simulink model "BaseEngineController_LS_112"  (Simulink 7.7)
settings: Solver=FixedStepDiscrete  StartTime=0.0  StopTime=10.0  RelTol=1e-3
PreLoadFcn:
  | try, eval([bdroot '_setup']); catch, eval('model_setup', ''); end
InitFcn:
  | try, eval([bdroot '_setup']); catch, eval('model_setup', ''); end
undefined symbols (not defined in the file): ECM, H1, H2, High, motohawk_build_version, motohawk_trunc_name, motohawk_vardec_config_group, motohawk_vardec_path, True, xD
libraries: MotoHawk_lib x1417, motohawk_control_primitives_lib x183, motohawk_engine_lib x32, simulink x21, motohawk_annotations_lib x9, AutoDoc_lib x8, simulink_extras x4, motohawk_ccp_examples_lib x1, motohawk_control_primitives_motoshare_lib x1
(part 5 of 27)

== system BaseEngineController_LS_112/Foreground/Control/Controller/Stall ==
  Inputs : Inport
  Enable : EnablePort  StatesWhenEnabling=reset
  Bus Creator2 : BusCreator  Inputs=13
  Data Type Conversion : DataTypeConversion  OutDataTypeStr=double
  Data Type Conversion1 : DataTypeConversion  OutDataTypeStr=double
  Data Type Conversion2 : DataTypeConversion  OutDataTypeStr=double
  FAN Control : Subsystem
  Fuel Pump at Startup : Subsystem
  No Fuel : Constant  Value=0
  No Spark : Constant  Value=0  OutDataTypeStr=Inherit: Inherit via back propagation
  No Spark Timing : Constant  Value=0  OutDataTypeStr=Inherit: Inherit via back propagation
  No Start EOI : Constant  Value=0
  No Start Fuel Timing : Constant  Value=0
  OFF{,1..3} (4 alike) : Constant  Value=0  OutDataTypeStr=boolean
  Stall Throttle : Subsystem
  Zero-Order Hold{1..9,11..14} (13 alike) : ZeroOrderHold  SampleTime=-1
  motohawk_replicate : MotoHawk_lib/Extra Development Blocks/motohawk_replicate  output_width=-1
  motohawk_replicate2 : MotoHawk_lib/Extra Development Blocks/motohawk_replicate  output_width=-1
  Actuators : Outport
  wires:
  Zero-Order Hold6/1 -> Bus Creator2/1  "FPC"
  No Spark/1 -> Zero-Order Hold4/1
  No Spark Timing/1 -> motohawk_replicate2/1
  No Fuel/1 -> motohawk_replicate/1
  Zero-Order Hold8/1 -> Bus Creator2/2  "SOI"
  No Start Fuel Timing/1 -> Zero-Order Hold8/1
  Bus Creator2/1 -> Actuators/1
  Stall Throttle/1(ETC %) -> Zero-Order Hold9/1
  Zero-Order Hold4/1 -> Bus Creator2/4  "SparkEnergy"
  Zero-Order Hold3/1 -> Bus Creator2/5  "SparkAdv"
  Zero-Order Hold9/1 -> Bus Creator2/6  "Throttle"
  Zero-Order Hold7/1 -> Bus Creator2/7  "FUELP"
  motohawk_replicate/1 -> Zero-Order Hold6/1
  Zero-Order Hold5/1 -> Bus Creator2/3  "EOI"
  No Start EOI/1 -> Zero-Order Hold5/1
  motohawk_replicate2/1 -> Zero-Order Hold3/1
  Fuel Pump at Startup/1(FUELP [bool]) -> Zero-Order Hold7/1
  OFF2/1 -> Zero-Order Hold1/1
  Zero-Order Hold1/1 -> Data Type Conversion2/1  "IAC-P"
  Zero-Order Hold2/1 -> Data Type Conversion1/1  "IAC-S"
  OFF/1 -> Zero-Order Hold11/1
  Zero-Order Hold11/1 -> Data Type Conversion/1  "WASTEGATE"
  OFF1/1 -> Zero-Order Hold2/1
  FAN Control/1(FAN-1) -> Zero-Order Hold12/1
  FAN Control/2(FAN-2) -> Zero-Order Hold13/1
  Inputs/1 -> FAN Control/1(Sensors), Stall Throttle/1(Sensors)
  OFF3/1 -> Zero-Order Hold14/1
  Data Type Conversion2/1 -> Bus Creator2/8  "IAC-P"
  Data Type Conversion1/1 -> Bus Creator2/9  "IAC-S"
  Data Type Conversion/1 -> Bus Creator2/10  "WASTEGATE"
  Zero-Order Hold12/1 -> Bus Creator2/11  "FAN-1"
  Zero-Order Hold13/1 -> Bus Creator2/12  "FAN-2"
  Zero-Order Hold14/1 -> Bus Creator2/13  "AC"

== system BaseEngineController_LS_112/Foreground/Control/Diagnostics/AC Fault ==
  Sensors : Inport
  Controller : Inport  Port=2
  Bus Selector1 : BusSelector  OutputSignals=Raw.LinearSensors.ACPres
  Bus Selector2 : BusSelector  OutputSignals=AC
  Logical Operator : Logic  Inputs=3  AllPortsSameDT=off  OutDataTypeStr=boolean
  Logical Operator1 : Logic  Inputs=4  AllPortsSameDT=off  OutDataTypeStr=boolean
  Logical Operator3 : Logic  Operator=OR  AllPortsSameDT=off  OutDataTypeStr=boolean
  Logical Operator4 : Logic  Operator=NOT  Inputs=3  AllPortsSameDT=off  OutDataTypeStr=boolean
  Relational Operator : RelationalOperator  OutDataTypeStr=boolean
  Relational Operator1 : RelationalOperator  Operator=<=  OutDataTypeStr=boolean
  Run State : motohawk_control_primitives_lib/CompareTo  SystemSampleTime=-1  op===  val=3
  motohawk_calibration : MotoHawk_lib/Calibration & Probing Blocks/motohawk_calibration  nam='ACHighPressureDisable'  val=3000  storage=Calibration  show_more=on  name_source=Use Parameter  data_type=uint16  read_level=1  write_level=1  ovr_cals=on  view_as=Number  enum_struct={'Disabled', 'Enabled'}  vector_style=Wide Row  use_help_units=on  help='Pressure when ac gets disabled'  units='kpa'  use_header_enum=off  row_header_enum={}  col_header_enum={}  use_min_max=off  min_val=-inf  max_val=inf  use_precision=off  precision=''  gain=1  offset=0  exp=1  use_mototune_group=off  mototune_group=motohawk_vardec_path(gcb)
  motohawk_calibration2 : MotoHawk_lib/Calibration & Probing Blocks/motohawk_calibration  nam='ACLowPressureDisable'  val=300  storage=Calibration  show_more=on  name_source=Use Parameter  data_type=uint16  read_level=1  write_level=1  ovr_cals=on  view_as=Number  enum_struct={'Disabled', 'Enabled'}  vector_style=Wide Row  use_help_units=on  help='Pressure when ac gets disabled'  units='kpa'  use_header_enum=off  row_header_enum={}  col_header_enum={}  use_min_max=off  min_val=-inf  max_val=inf  use_precision=off  precision=''  gain=1  offset=0  exp=1  use_mototune_group=off  mototune_group=motohawk_vardec_path(gcb)
  motohawk_data_read : MotoHawk_lib/Data Storage Blocks/motohawk_data_read  source=Lookup By Name  structure=Scalar  operation=Read entire data structure at once  sz_vec=4  sz_row=2  sz_col=3  typ=uint8  nam='EngineState'  checkNull=on  struct_inst_name='Struct1'  struct_nam='MyStruct'
  motohawk_fault_def1 : MotoHawk_lib/Fault Management Blocks/motohawk_fault_def  nam='ACChargeHigh_Fault'  mode=Enabled  id=[]  x=25  y=50  input_suspected=on  indeterminate=off  increment_xy=on  downsample_count=1  ovr_cals=on  ovr_actions=on  show_actions=on  action1_name='DisableAC'  action1_cond=Active  action2_name=''  action2_cond=(None)  action3_name=''  action3_cond=(None)  action4_name=''  action4_cond=(None)
  motohawk_fault_def2 : MotoHawk_lib/Fault Management Blocks/motohawk_fault_def  nam='ACChargeLow_Fault'  mode=Enabled  id=[]  x=25  y=50  input_suspected=on  indeterminate=off  increment_xy=on  downsample_count=1  ovr_cals=on  ovr_actions=on  show_actions=on  action1_name='DisableAC'  action1_cond=Active  action2_name=''  action2_cond=(None)  action3_name=''  action3_cond=(None)  action4_name=''  action4_cond=(None)
  motohawk_fault_status1 : MotoHawk_lib/Fault Management Blocks/motohawk_fault_status  source=Lookup By Name  nam='ACPresRangeHigh'  status=Active
  motohawk_fault_status4 : MotoHawk_lib/Fault Management Blocks/motohawk_fault_status  source=Lookup By Name  nam='ACPresRangeLow'  status=Active
  wires:
  Sensors/1 -> Bus Selector1/1
  motohawk_data_read/1 -> Run State/1
  Logical Operator/1 -> motohawk_fault_def1/1
  Logical Operator1/1 -> motohawk_fault_def2/1
  Controller/1 -> Bus Selector2/1
  Relational Operator/1 -> Logical Operator/2
  Bus Selector1/1 -> Relational Operator/1, Relational Operator1/1  "<ACPres>"
  motohawk_calibration/1 -> Relational Operator/2
  motohawk_calibration2/1 -> Relational Operator1/2
  Relational Operator1/1 -> Logical Operator1/2
  motohawk_fault_status1/1 -> Logical Operator3/1
  Logical Operator3/1 -> Logical Operator4/1
  motohawk_fault_status4/1 -> Logical Operator3/2
  Bus Selector2/1 -> Logical Operator1/4  "<AC>"
  Run State/1 -> Logical Operator/1, Logical Operator1/1
  Logical Operator4/1 -> Logical Operator/3, Logical Operator1/3

== system BaseEngineController_LS_112/Foreground/Control/Diagnostics/AirFlow ==
  Sensors : Inport
  Abs : Abs
  Bus Selector1 : BusSelector  OutputSignals=RawIndexes.RPM09Idx,RawIndexes.MAP09Idx
  Bus Selector4 : BusSelector  OutputSignals=Raw.Digital.MAF
  Logical Operator1 : Logic  Operator=NOT  Inputs=3  AllPortsSameDT=off  OutDataTypeStr=boolean
  Logical Operator2 : Logic  Operator=OR  Inputs=4  AllPortsSameDT=off  OutDataTypeStr=boolean
  Logical Operator3 : Logic  Operator=OR  Inputs=4  AllPortsSameDT=off  OutDataTypeStr=boolean
  Logical Operator4 : Logic  Inputs=3  AllPortsSameDT=off  OutDataTypeStr=boolean
  Logical Operator5 : Logic  Operator=OR  Inputs=3  AllPortsSameDT=off  OutDataTypeStr=boolean
  Logical Operator6 : Logic  Operator=NOT  Inputs=3  AllPortsSameDT=off  OutDataTypeStr=boolean
  Logical Operator7 : Logic  AllPortsSameDT=off  OutDataTypeStr=boolean
  Logical Operator8 : Logic  Inputs=3  AllPortsSameDT=off  OutDataTypeStr=boolean
  Logical Operator9 : Logic  Operator=NOT  Inputs=3  AllPortsSameDT=off  OutDataTypeStr=boolean
  Relational Operator : RelationalOperator  OutDataTypeStr=boolean
  Run State : motohawk_control_primitives_lib/CompareTo  SystemSampleTime=-1  op===  val=3
  Sum : Sum  Inputs=|+-
  motohawk_calibration3 : MotoHawk_lib/Calibration & Probing Blocks/motohawk_calibration  nam='AirflowDiag_MAPIRDiagEnable'  val=0  storage=Calibration  show_more=on  name_source=Use Parameter  data_type=boolean  read_level=1  write_level=1  ovr_cals=on  view_as=Enumeration  enum_struct={'Disabled', 'Enabled'}  vector_style=Wide Row  use_help_units=off  help=''  units=''  use_header_enum=off  row_header_enum={}  col_header_enum={}  use_min_max=off  min_val=-inf  max_val=inf  use_precision=off  precision=''  gain=1  offset=0  exp=1  use_mototune_group=off  mototune_group=motohawk_vardec_path(gcb)
  motohawk_data_read : MotoHawk_lib/Data Storage Blocks/motohawk_data_read  source=Lookup By Name  structure=Scalar  operation=Read scalar from location by index  sz_vec=4  sz_row=2  sz_col=3  typ=double  nam='VEModelMAF'  checkNull=on  struct_inst_name='MyData'  struct_nam='MyStruct'
  motohawk_data_read1 : MotoHawk_lib/Data Storage Blocks/motohawk_data_read  source=Lookup By Name  structure=Scalar  operation=Read entire data structure at once  sz_vec=4  sz_row=2  sz_col=3  typ=uint8  nam='EngineState'  checkNull=on  struct_inst_name='Struct1'  struct_nam='MyStruct'
  motohawk_fault_def1 : MotoHawk_lib/Fault Management Blocks/motohawk_fault_def  nam='AirflowMismatch_Fault'  mode=Enabled  id=[]  x=25  y=50  input_suspected=on  indeterminate=off  increment_xy=on  downsample_count=1  ovr_cals=on  ovr_actions=on  show_actions=on  action1_name=''  action1_cond=(None)  action2_name=''  action2_cond=(None)  action3_name=''  action3_cond=(None)  action4_name=''  action4_cond=(None)
  motohawk_fault_status1 : MotoHawk_lib/Fault Management Blocks/motohawk_fault_status  source=Lookup By Name  nam='MAPRangeHigh'  status=Active
  motohawk_fault_status10 : MotoHawk_lib/Fault Management Blocks/motohawk_fault_status  source=Lookup By Name  nam='CamSyncFault'  status=Active
  motohawk_fault_status11 : MotoHawk_lib/Fault Management Blocks/motohawk_fault_status  source=Lookup By Name  nam='CrankEdgesFault'  status=Active
  motohawk_fault_status2 : MotoHawk_lib/Fault Management Blocks/motohawk_fault_status  source=Lookup By Name  nam='MAP_IR_HI'  status=Active
  motohawk_fault_status3 : MotoHawk_lib/Fault Management Blocks/motohawk_fault_status  source=Lookup By Name  nam='MAP_IR_LO'  status=Active
  motohawk_fault_status4 : MotoHawk_lib/Fault Management Blocks/motohawk_fault_status  source=Lookup By Name  nam='MAPRangeLow'  status=Active
  motohawk_fault_status5 : MotoHawk_lib/Fault Management Blocks/motohawk_fault_status  source=Lookup By Name  nam='MAP_STICKING'  status=Active
  motohawk_fault_status6 : MotoHawk_lib/Fault Management Blocks/motohawk_fault_status  source=Lookup By Name  nam='MAFRangeHigh'  status=Active
  motohawk_fault_status7 : MotoHawk_lib/Fault Management Blocks/motohawk_fault_status  source=Lookup By Name  nam='MAFRangeLow'  status=Active
  motohawk_fault_status8 : MotoHawk_lib/Fault Management Blocks/motohawk_fault_status  source=Lookup By Name  nam='CrankSyncFault'  status=Active
  motohawk_fault_status9 : MotoHawk_lib/Fault Management Blocks/motohawk_fault_status  source=Lookup By Name  nam='CamEdgesFault'  status=Active
  motohawk_interpolation_2d : MotoHawk_lib/Lookup Tables/motohawk_interpolation_2d  nam='AirflowMimatchThresh'  table_data=zeros(9,9)  show_more=on  data_type=int8  storage=NonAdaptive  read_level=1  write_level=1  ovr_cals=on  use_help=off  help=''  units=''  use_min_max=off  min_val=-inf  max_val=inf  use_precision=off  precision=''  gain=1  offset=0  exp=1  use_links=off  row_prelookup_block=''  col_prelookup_block=''  output_name=''  use_mototune_group=off  mototune_group=motohawk_vardec_path(gcb)
  wires:
  Sensors/1 -> Bus Selector4/1, Bus Selector1/1
  motohawk_data_read1/1 -> Run State/1
  Run State/1 -> Logical Operator4/3
  Logical Operator4/1 -> motohawk_fault_def1/1
  Bus Selector4/1 -> Sum/1  "<MAF>"
  motohawk_data_read/1 -> Sum/2
  Sum/1 -> Abs/1
  Abs/1 -> Relational Operator/1
  Bus Selector1/1 -> motohawk_interpolation_2d/1  "<RPM09Idx>"
  Bus Selector1/2 -> motohawk_interpolation_2d/2  "<MAP09Idx>"
  motohawk_interpolation_2d/1 -> Relational Operator/2
  Relational Operator/1 -> Logical Operator4/2
  motohawk_fault_status1/1 -> Logical Operator3/1
  Logical Operator3/1 -> Logical Operator1/1
  motohawk_fault_status4/1 -> Logical Operator3/2
  motohawk_fault_status2/1 -> Logical Operator5/1
  motohawk_fault_status3/1 -> Logical Operator5/2
  motohawk_fault_status5/1 -> Logical Operator5/3
  Logical Operator5/1 -> Logical Operator7/1
  motohawk_calibration3/1 -> Logical Operator7/2
  Logical Operator7/1 -> Logical Operator6/1
  Logical Operator1/1 -> Logical Operator8/1
  Logical Operator6/1 -> Logical Operator8/2
  motohawk_fault_status6/1 -> Logical Operator3/3
  motohawk_fault_status7/1 -> Logical Operator3/4
  motohawk_fault_status8/1 -> Logical Operator2/1
  Logical Operator2/1 -> Logical Operator9/1
  motohawk_fault_status11/1 -> Logical Operator2/2
  motohawk_fault_status9/1 -> Logical Operator2/3
  motohawk_fault_status10/1 -> Logical Operator2/4
  Logical Operator9/1 -> Logical Operator8/3
  Logical Operator8/1 -> Logical Operator4/1

== system BaseEngineController_LS_112/Foreground/Control/Diagnostics/Boost Fault ==
  note: BOOST Level
  Sensors : Inport
  Controller : Inport  Port=2
  Bus Selector1 : BusSelector  OutputSignals=Raw.LinearSensors.MAP_Angular
  Bus Selector2 : BusSelector  OutputSignals=WASTEGATE
  Logical Operator : Logic  Inputs=3  AllPortsSameDT=off  OutDataTypeStr=boolean
  Logical Operator1 : Logic  Inputs=3  AllPortsSameDT=off  OutDataTypeStr=boolean
  Logical Operator2 : Logic  Inputs=3  AllPortsSameDT=off  OutDataTypeStr=boolean
  Logical Operator3 : Logic  Operator=OR  AllPortsSameDT=off  OutDataTypeStr=boolean
  Logical Operator4 : Logic  Operator=NOT  Inputs=3  AllPortsSameDT=off  OutDataTypeStr=boolean
  Logical Operator5 : Logic  Operator=OR  Inputs=3  AllPortsSameDT=off  OutDataTypeStr=boolean
  Logical Operator6 : Logic  Operator=NOT  Inputs=3  AllPortsSameDT=off  OutDataTypeStr=boolean
  Logical Operator7 : Logic  AllPortsSameDT=off  OutDataTypeStr=boolean
  Logical Operator8 : Logic  AllPortsSameDT=off  OutDataTypeStr=boolean
  Relational Operator : RelationalOperator  OutDataTypeStr=boolean
  Relational Operator1 : RelationalOperator  OutDataTypeStr=boolean
  Relational Operator2 : RelationalOperator  OutDataTypeStr=boolean
  Run State : motohawk_control_primitives_lib/CompareTo  SystemSampleTime=-1  op===  val=3
  kPa to PSI : Gain  Gain=0.145038
  motohawk_calibration : MotoHawk_lib/Calibration & Probing Blocks/motohawk_calibration  nam='SoftOverBoostLimit'  val=20  storage=Calibration  show_more=on  name_source=Use Parameter  data_type=Inherit from 'Default Value'  read_level=1  write_level=1  ovr_cals=on  view_as=Number  enum_struct={'Disabled', 'Enabled'}  vector_style=Wide Row  use_help_units=on  help='Soft overboost limit'  units='PSI'  use_header_enum=off  row_header_enum={}  col_header_enum={}  use_min_max=off  min_val=-inf  max_val=inf  use_precision=off  precision=''  gain=1  offset=0  exp=1  use_mototune_group=off  mototune_group=motohawk_vardec_path(gcb)
  motohawk_calibration1 : MotoHawk_lib/Calibration & Probing Blocks/motohawk_calibration  nam='HardOverBoostLimit'  val=25  storage=Calibration  show_more=on  name_source=Use Parameter  data_type=Inherit from 'Default Value'  read_level=1  write_level=1  ovr_cals=on  view_as=Number  enum_struct={'Disabled', 'Enabled'}  vector_style=Wide Row  use_help_units=on  help='Hard overboost limit'  units='PSI'  use_header_enum=off  row_header_enum={}  col_header_enum={}  use_min_max=off  min_val=-inf  max_val=inf  use_precision=off  precision=''  gain=1  offset=0  exp=1  use_mototune_group=off  mototune_group=motohawk_vardec_path(gcb)
  motohawk_calibration2 : MotoHawk_lib/Calibration & Probing Blocks/motohawk_calibration  nam='WastegateLossOfControl'  val=50  storage=Calibration  show_more=on  name_source=Use Parameter  data_type=Inherit from 'Default Value'  read_level=1  write_level=1  ovr_cals=on  view_as=Number  enum_struct={'Disabled', 'Enabled'}  vector_style=Wide Row  use_help_units=on  help='Wastegate duty cycle having insufficient control of boost'  units='%'  use_header_enum=off  row_header_enum={}  col_header_enum={}  use_min_max=off  min_val=-inf  max_val=inf  use_precision=off  precision=''  gain=1  offset=0  exp=1  use_mototune_group=off  mototune_group=motohawk_vardec_path(gcb)
  motohawk_calibration3 : MotoHawk_lib/Calibration & Probing Blocks/motohawk_calibration  nam='BoostDiag_MAPIRDiagEnable'  val=0  storage=Calibration  show_more=on  name_source=Use Parameter  data_type=boolean  read_level=1  write_level=1  ovr_cals=on  view_as=Enumeration  enum_struct={'Disabled', 'Enabled'}  vector_style=Wide Row  use_help_units=off  help=''  units=''  use_header_enum=off  row_header_enum={}  col_header_enum={}  use_min_max=off  min_val=-inf  max_val=inf  use_precision=off  precision=''  gain=1  offset=0  exp=1  use_mototune_group=off  mototune_group=motohawk_vardec_path(gcb)
  motohawk_data_read : MotoHawk_lib/Data Storage Blocks/motohawk_data_read  source=Lookup By Name  structure=Scalar  operation=Read entire data structure at once  sz_vec=4  sz_row=2  sz_col=3  typ=uint8  nam='EngineState'  checkNull=on  struct_inst_name='Struct1'  struct_nam='MyStruct'
  motohawk_fault_def1 : MotoHawk_lib/Fault Management Blocks/motohawk_fault_def  nam='SoftOverBoost_Fault'  mode=Sticky  id=[]  x=1  y=2  input_suspected=on  indeterminate=off  increment_xy=on  downsample_count=1  ovr_cals=on  ovr_actions=on  show_actions=on  action1_name='EngineShutdown'  action1_cond=(None)  action2_name='DisableWastegate'  action2_cond=(None)  action3_name=''  action3_cond=(None)  action4_name=''  action4_cond=(None)
  motohawk_fault_def2 : MotoHawk_lib/Fault Management Blocks/motohawk_fault_def  nam='HardOverBoost_Fault'  mode=Sticky  id=[]  x=1  y=2  input_suspected=on  indeterminate=off  increment_xy=on  downsample_count=1  ovr_cals=on  ovr_actions=on  show_actions=on  action1_name='EngineShutdown'  action1_cond=(None)  action2_name='DisableWastegate'  action2_cond=(None)  action3_name=''  action3_cond=(None)  action4_name=''  action4_cond=(None)
  motohawk_fault_def3 : MotoHawk_lib/Fault Management Blocks/motohawk_fault_def  nam='Wastegate_Fault'  mode=Sticky  id=[]  x=1  y=2  input_suspected=on  indeterminate=off  increment_xy=on  downsample_count=1  ovr_cals=on  ovr_actions=on  show_actions=on  action1_name='EngineShutdown'  action1_cond=(None)  action2_name='DisableWastegate'  action2_cond=(None)  action3_name=''  action3_cond=(None)  action4_name=''  action4_cond=(None)
  motohawk_fault_status1 : MotoHawk_lib/Fault Management Blocks/motohawk_fault_status  source=Lookup By Name  nam='MAPRangeHigh'  status=Active
  motohawk_fault_status2 : MotoHawk_lib/Fault Management Blocks/motohawk_fault_status  source=Lookup By Name  nam='MAP_IR_HI'  status=Active
  motohawk_fault_status3 : MotoHawk_lib/Fault Management Blocks/motohawk_fault_status  source=Lookup By Name  nam='MAP_IR_LO'  status=Active
  motohawk_fault_status4 : MotoHawk_lib/Fault Management Blocks/motohawk_fault_status  source=Lookup By Name  nam='MAPRangeLow'  status=Active
  motohawk_fault_status5 : MotoHawk_lib/Fault Management Blocks/motohawk_fault_status  source=Lookup By Name  nam='MAP_STICKING'  status=Active
  wires:
  Sensors/1 -> Bus Selector1/1
  motohawk_data_read/1 -> Run State/1
  kPa to PSI/1 -> Relational Operator/1, Relational Operator1/1
  Controller/1 -> Bus Selector2/1
  Bus Selector2/1 -> Relational Operator2/1  "<WASTEGATE>"
  motohawk_calibration/1 -> Relational Operator/2
  motohawk_calibration1/1 -> Relational Operator1/2
  motohawk_calibration2/1 -> Relational Operator2/2
  Relational Operator/1 -> Logical Operator/2
  Logical Operator/1 -> motohawk_fault_def1/1
  Logical Operator1/1 -> motohawk_fault_def2/1
  Relational Operator1/1 -> Logical Operator1/2
  Logical Operator2/1 -> motohawk_fault_def3/1
  Relational Operator2/1 -> Logical Operator2/2
  Bus Selector1/1 -> kPa to PSI/1  "<MAP_Angular>"
  motohawk_fault_status1/1 -> Logical Operator3/1
  Logical Operator3/1 -> Logical Operator4/1
  motohawk_fault_status4/1 -> Logical Operator3/2
  motohawk_fault_status2/1 -> Logical Operator5/1
  motohawk_fault_status3/1 -> Logical Operator5/2
  motohawk_fault_status5/1 -> Logical Operator5/3
  Logical Operator5/1 -> Logical Operator7/1
  motohawk_calibration3/1 -> Logical Operator7/2
  Logical Operator7/1 -> Logical Operator6/1
  Logical Operator4/1 -> Logical Operator8/1
  Logical Operator6/1 -> Logical Operator8/2
  Run State/1 -> Logical Operator/1, Logical Operator1/1, Logical Operator2/1
  Logical Operator8/1 -> Logical Operator/3, Logical Operator1/3, Logical Operator2/3

== system BaseEngineController_LS_112/Foreground/Control/Diagnostics/Digital Sensors ==
  Sensors : Inport
  Bus Selector1 : BusSelector  OutputSignals=Raw.Digital.Scramble
  Bus Selector2 : BusSelector  OutputSignals=Raw.Digital.ClutchSw
  Logical Operator1 : Logic  AllPortsSameDT=off  OutDataTypeStr=boolean
  Logical Operator2 : Logic  AllPortsSameDT=off  OutDataTypeStr=boolean
  Relational Operator1 : RelationalOperator  OutDataTypeStr=boolean
  Relational Operator2 : RelationalOperator  OutDataTypeStr=boolean
  Time Since Enabled (With Input)2 : motohawk_control_primitives_lib/Time Since Enabled (With Input)1  SystemSampleTime=-1  nam='ScrambleTime'  samp_time=-1  init=0  upperlim=16000
  Time Since Enabled (With Input)3 : motohawk_control_primitives_lib/Time Since Enabled (With Input)1  SystemSampleTime=-1  nam='ClutchTime'  samp_time=-1  init=0  upperlim=16000
  motohawk_calibration1 : MotoHawk_lib/Calibration & Probing Blocks/motohawk_calibration  nam='DigDiag_ScrambleStuckTime'  val=30  storage=Calibration  show_more=off  name_source=Use Parameter  data_type=Inherit from 'Default Value'  read_level=1  write_level=1  ovr_cals=on  view_as=Number  enum_struct={'Disabled', 'Enabled'}  vector_style=Wide Row  use_help_units=off  help=''  units=''  use_header_enum=off  row_header_enum={}  col_header_enum={}  use_min_max=off  min_val=-inf  max_val=inf  use_precision=off  precision=''  gain=1  offset=0  exp=1  use_mototune_group=off  mototune_group=motohawk_vardec_path(gcb)
  motohawk_calibration2 : MotoHawk_lib/Calibration & Probing Blocks/motohawk_calibration  nam='DigDiag_ClutchStuckTime'  val=30  storage=Calibration  show_more=off  name_source=Use Parameter  data_type=Inherit from 'Default Value'  read_level=1  write_level=1  ovr_cals=on  view_as=Number  enum_struct={'Disabled', 'Enabled'}  vector_style=Wide Row  use_help_units=off  help=''  units=''  use_header_enum=off  row_header_enum={}  col_header_enum={}  use_min_max=off  min_val=-inf  max_val=inf  use_precision=off  precision=''  gain=1  offset=0  exp=1  use_mototune_group=off  mototune_group=motohawk_vardec_path(gcb)
  motohawk_fault_def2 : MotoHawk_lib/Fault Management Blocks/motohawk_fault_def  nam='ScrambleStuckHigh_Fault'  mode=Enabled  id=[]  x=25  y=50  input_suspected=on  indeterminate=off  increment_xy=on  downsample_count=1  ovr_cals=on  ovr_actions=on  show_actions=on  action1_name=''  action1_cond=(None)  action2_name=''  action2_cond=(None)  action3_name=''  action3_cond=(None)  action4_name=''  action4_cond=(None)
  motohawk_fault_def3 : MotoHawk_lib/Fault Management Blocks/motohawk_fault_def  nam='ClutchStuckHigh_Fault'  mode=Enabled  id=[]  x=25  y=50  input_suspected=on  indeterminate=off  increment_xy=on  downsample_count=1  ovr_cals=on  ovr_actions=on  show_actions=on  action1_name=''  action1_cond=(None)  action2_name=''  action2_cond=(None)  action3_name=''  action3_cond=(None)  action4_name=''  action4_cond=(None)
  wires:
  Sensors/1 -> Bus Selector1/1, Bus Selector2/1
  Time Since Enabled (With Input)2/1 -> Relational Operator1/1
  motohawk_calibration1/1 -> Relational Operator1/2
  Bus Selector1/1 -> Time Since Enabled (With Input)2/1, Logical Operator1/2  "<Scramble>"
  Time Since Enabled (With Input)3/1 -> Relational Operator2/1
  motohawk_calibration2/1 -> Relational Operator2/2
  Bus Selector2/1 -> Time Since Enabled (With Input)3/1, Logical Operator2/2  "<ClutchSw>"
  Relational Operator1/1 -> Logical Operator1/1
  Relational Operator2/1 -> Logical Operator2/1
  Logical Operator2/1 -> motohawk_fault_def3/1
  Logical Operator1/1 -> motohawk_fault_def2/1

== system BaseEngineController_LS_112/Foreground/Control/Diagnostics/Engine Overheat Fault Logic ==
  Sensors : Inport
  Bus Selector : BusSelector  OutputSignals=Raw.NonLinearSensors.ECT
  Logical Operator1 : Logic  Operator=OR  AllPortsSameDT=off  OutDataTypeStr=boolean
  Logical Operator2 : Logic  Inputs=3  AllPortsSameDT=off  OutDataTypeStr=boolean
  Logical Operator3 : Logic  Operator=NOT  Inputs=3  AllPortsSameDT=off  OutDataTypeStr=boolean
  Logical Operator4 : Logic  Inputs=3  AllPortsSameDT=off  OutDataTypeStr=boolean
  Relational Operator1 : RelationalOperator  OutDataTypeStr=boolean
  Relational Operator2 : RelationalOperator  OutDataTypeStr=boolean
  Relational Operator3 : RelationalOperator  OutDataTypeStr=boolean
  Run State : motohawk_control_primitives_lib/CompareTo  SystemSampleTime=-1  op===  val=3
  motohawk_calibration1 : MotoHawk_lib/Calibration & Probing Blocks/motohawk_calibration  nam='TempOverheat_Warn'  val=95  storage=Calibration  show_more=on  name_source=Use Parameter  data_type=double  read_level=1  write_level=1  ovr_cals=on  view_as=Number  enum_struct={'Disabled', 'Enabled'}  vector_style=Wide Row  use_help_units=on  help='ECT limit above which warning light comes on'  units='degC'  use_header_enum=off  row_header_enum={}  col_header_enum={}  use_min_max=off  min_val=-inf  max_val=inf  use_precision=off  precision=''  gain=1  offset=0  exp=1  use_mototune_group=on  mototune_group=motohawk_vardec_path(gcb)
  motohawk_calibration2 : MotoHawk_lib/Calibration & Probing Blocks/motohawk_calibration  nam='TempOverheat_Fault'  val=100  storage=Calibration  show_more=on  name_source=Use Parameter  data_type=double  read_level=1  write_level=1  ovr_cals=on  view_as=Number  enum_struct={'Disabled', 'Enabled'}  vector_style=Wide Row  use_help_units=on  help='ECT limit above which fault is set.'  units='degC'  use_header_enum=off  row_header_enum={}  col_header_enum={}  use_min_max=off  min_val=-inf  max_val=inf  use_precision=off  precision=''  gain=1  offset=0  exp=1  use_mototune_group=on  mototune_group=motohawk_vardec_path(gcb)
  motohawk_calibration3 : MotoHawk_lib/Calibration & Probing Blocks/motohawk_calibration  nam='TempOverheatSevere_Fault'  val=110  storage=Calibration  show_more=on  name_source=Use Parameter  data_type=double  read_level=1  write_level=1  ovr_cals=on  view_as=Number  enum_struct={'Disabled', 'Enabled'}  vector_style=Wide Row  use_help_units=on  help='ECT limit above which severe overheat fault is set.'  units='degC'  use_header_enum=off  row_header_enum={}  col_header_enum={}  use_min_max=off  min_val=-inf  max_val=inf  use_precision=off  precision=''  gain=1  offset=0  exp=1  use_mototune_group=on  mototune_group=motohawk_vardec_path(gcb)
  motohawk_data_read : MotoHawk_lib/Data Storage Blocks/motohawk_data_read  source=Lookup By Name  structure=Scalar  operation=Read entire data structure at once  sz_vec=4  sz_row=2  sz_col=3  typ=uint8  nam='EngineState'  checkNull=on  struct_inst_name='Struct1'  struct_nam='MyStruct'
  motohawk_fault_def1 : MotoHawk_lib/Fault Management Blocks/motohawk_fault_def  nam='ECTOverTempFault'  mode=Enabled  id=[]  x=25  y=50  input_suspected=on  indeterminate=off  increment_xy=on  downsample_count=1  ovr_cals=on  ovr_actions=on  show_actions=off  action1_name=''  action1_cond=(None)  action2_name=''  action2_cond=(None)  action3_name=''  action3_cond=(None)  action4_name=''  action4_cond=(None)
  motohawk_fault_def2 : MotoHawk_lib/Fault Management Blocks/motohawk_fault_def  nam='ECTSevereOverTempFault'  mode=Enabled  id=[]  x=25  y=50  input_suspected=on  indeterminate=off  increment_xy=on  downsample_count=1  ovr_cals=on  ovr_actions=on  show_actions=off  action1_name=''  action1_cond=(None)  action2_name=''  action2_cond=(None)  action3_name=''  action3_cond=(None)  action4_name=''  action4_cond=(None)
  motohawk_fault_status : MotoHawk_lib/Fault Management Blocks/motohawk_fault_status  source=Lookup By Name  nam='ECTRangeHigh'  status=Active
  motohawk_fault_status1 : MotoHawk_lib/Fault Management Blocks/motohawk_fault_status  source=Lookup By Name  nam='ECTRangeLow'  status=Active
  Overheat_Warning : Outport
  wires:
  motohawk_data_read/1 -> Run State/1
  Bus Selector/1 -> Relational Operator3/1, Relational Operator1/1, Relational Operator2/1  "<ECT>"
  motohawk_calibration2/1 -> Relational Operator3/2
  Sensors/1 -> Bus Selector/1
  Relational Operator3/1 -> Logical Operator2/3
  Logical Operator2/1 -> motohawk_fault_def1/1
  Run State/1 -> Logical Operator2/2, Logical Operator4/2
  motohawk_fault_status/1 -> Logical Operator1/1
  motohawk_fault_status1/1 -> Logical Operator1/2
  Logical Operator1/1 -> Logical Operator3/1
  Logical Operator3/1 -> Logical Operator2/1, Logical Operator4/1
  motohawk_calibration1/1 -> Relational Operator1/2
  Relational Operator1/1 -> Overheat_Warning/1
  motohawk_calibration3/1 -> Relational Operator2/2
  Relational Operator2/1 -> Logical Operator4/3
  Logical Operator4/1 -> motohawk_fault_def2/1

== system BaseEngineController_LS_112/Foreground/Control/Diagnostics/Fuel Economy ==
  Sensors : Inport
  Controller : Inport  Port=2
  Bus Selector1 : BusSelector  OutputSignals=FPC
  Bus Selector2 : BusSelector  OutputSignals=Raw.RPM
  Bus Selector3 : BusSelector  OutputSignals=Raw.LinearSensors.FuelSense
  Bus Selector4 : BusSelector  OutputSignals=RawProcessed.VSPD_Final
  Calculate Fuel Density : Subsystem
  Constant1 : Constant
  Constant2 : Constant
  Data Type Conversion : DataTypeConversion  SaturateOnIntegerOverflow=on  RndMeth=Zero
  Default (if no flow) : Switch  Threshold=0.5  ZeroCross=off  SaturateOnIntegerOverflow=on  InputSameDT=on
  Default value : Constant  Value=0
  First Order Low Pass (Tunable) : Subsystem  AncestorBlock=motohawk_control_primitives_lib/First Order Low Pass (Tunable)  mask(First-Order Low-Pass Filter (Tunable)){nam='FuelEconomy_Filter', samp_time=-1, group=motohawk_vardec_path(gcb)}
      mask prompts: nam "Name"; samp_time "Sample Time"; group "MotoTune Group String"
      mask help:
      | Discrete first-order low-pass filter, with calibratable time-constant.
      |
      | If 'Sample Time' is -1, then extra code and RAM will be generated to dynamically calculate dt.
      mask Display:
      | patch([0 0 1 1], [0 0.075 0.075 0], [230/255 0/255 0/255])
      | patch([0 0 1 1], [0.025 0.05 0.05 0.025], [150/255 0/255 0/255])
      | patch([0 0 1 1], [0 0.025 0.025 0], [0/255 0/255 0/255])
      | 
      | disp('1st-Order\nLow Pass');
  Mass flow to Volume flow mg/hr to ml/hr : Product  Inputs=*/  SaturateOnIntegerOverflow=on  InputSameDT=on  OutDataTypeStr=Inherit: Same as first input
  Min fuel flow  for calc : Constant  Value=0.1
  "Multiply and Divide, avoiding divde by zero1" : motohawk_engine_lib/Mass Flow to Charge Mass Transform/Multiply and Divide, avoiding divde by zero  SystemSampleTime=-1
  Number of Combustion Events Per Revolution : MotoHawk_lib/Data Storage Blocks/motohawk_data_read  source=Lookup By Name  structure=Scalar  operation=Read scalar from location by index  sz_vec=-1  sz_row=-1  sz_col=-1  typ=uint8  nam='CombEventsPerRev'  checkNull=on  struct_inst_name='Struct1'  struct_nam='MyStruct'
  RPM to inj/min : Product  RndMeth=Zero
  Relational Operator7 : RelationalOperator  Operator=>  OutDataTypeStr=boolean
  g to mg : Gain  Gain=1000
  inj/hr to mg/hr : Product  RndMeth=Zero
  inj/min to inj/hr : Gain  Gain=60
  ml/hr to gal/hr : Gain  Gain=1/3785.41178
  motohawk_probe : MotoHawk_lib/Calibration & Probing Blocks/motohawk_probe  nam='Fuel_Economy_Inst'  show_more=off  name_source=Use Parameter  read_level=1  view_as=Number  enum_struct={'Disabled', 'Enabled'}  vector_style=Wide Row  use_help_units=off  help=''  units=''  use_header_enum=off  row_header_enum={}  col_header_enum={}  use_precision=off  precision=''  gain=1  offset=0  exp=1  use_mototune_group=off  mototune_group=motohawk_vardec_path(gcb)
  motohawk_probe1 : MotoHawk_lib/Calibration & Probing Blocks/motohawk_probe  nam='Fuel_Economy_Filtered'  show_more=off  name_source=Use Parameter  read_level=1  view_as=Number  enum_struct={'Disabled', 'Enabled'}  vector_style=Wide Row  use_help_units=off  help=''  units=''  use_header_enum=off  row_header_enum={}  col_header_enum={}  use_precision=off  precision=''  gain=1  offset=0  exp=1  use_mototune_group=off  mototune_group=motohawk_vardec_path(gcb)
  FuelEconomy_instantaneous : Outport
  FuelEconomy_filtered : Outport  Port=2
  wires:
  Sensors/1 -> Bus Selector2/1, Bus Selector3/1, Bus Selector4/1
  Controller/1 -> Bus Selector1/1
  Bus Selector2/1 -> RPM to inj/min/1  "<RPM>"
  Number of Combustion Events Per Revolution/1 -> Data Type Conversion/1
  RPM to inj/min/1 -> inj/min to inj/hr/1
  inj/min to inj/hr/1 -> inj/hr to mg/hr/1
  Bus Selector1/1 -> inj/hr to mg/hr/2  "<FPC>"
  Bus Selector3/1 -> Calculate Fuel Density/1(Ethanol_xx [%])  "<FuelSense>"
  Calculate Fuel Density/1(Fuel Density (g/ml)) -> g to mg/1
  Data Type Conversion/1 -> RPM to inj/min/2
  inj/hr to mg/hr/1 -> Mass flow to Volume flow mg/hr to ml/hr/1
  g to mg/1 -> Mass flow to Volume flow mg/hr to ml/hr/2
  Mass flow to Volume flow mg/hr to ml/hr/1 -> ml/hr to gal/hr/1
  Constant2/1 -> "Multiply and Divide, avoiding divde by zero1"/2
  Constant1/1 -> "Multiply and Divide, avoiding divde by zero1"/4
  ml/hr to gal/hr/1 -> "Multiply and Divide, avoiding divde by zero1"/3, Relational Operator7/1
  Min fuel flow  for calc/1 -> Relational Operator7/2
  Relational Operator7/1 -> "Multiply and Divide, avoiding divde by zero1"/Enable, Default (if no flow)/2
  "Multiply and Divide, avoiding divde by zero1"/1 -> Default (if no flow)/1
  Default value/1 -> Default (if no flow)/3
  Default (if no flow)/1 -> First Order Low Pass (Tunable)/1(in), FuelEconomy_instantaneous/1, motohawk_probe/1
  First Order Low Pass (Tunable)/1(out) -> FuelEconomy_filtered/1, motohawk_probe1/1
  Bus Selector4/1 -> "Multiply and Divide, avoiding divde by zero1"/1  "<VSPD_Final>"

== system BaseEngineController_LS_112/Foreground/Control/Diagnostics/Lean Protect ==
  Sensors : Inport
  Bus Selector1 : BusSelector  OutputSignals=Raw.Digital.ESTOP
  Bus Selector4 : BusSelector  OutputSignals=Raw.CAN.O2_BankA
  Logical Operator1 : Logic  Operator=OR  Inputs=5  AllPortsSameDT=off  OutDataTypeStr=boolean
  Logical Operator3 : Logic  Operator=NOT  Inputs=3  AllPortsSameDT=off  OutDataTypeStr=boolean
  Logical Operator4 : Logic  Inputs=3  AllPortsSameDT=off  OutDataTypeStr=boolean
  Product : Product  RndMeth=Zero
  Product1 : Product  RndMeth=Zero
  Relational Operator1 : RelationalOperator  Operator=<  OutDataTypeStr=boolean
  Run State : motohawk_control_primitives_lib/CompareTo  SystemSampleTime=-1  op===  val=3
  motohawk_calibration3 : MotoHawk_lib/Calibration & Probing Blocks/motohawk_calibration  nam='LeanProtect_Threshold'  val=0.85  storage=Calibration  show_more=on  name_source=Use Parameter  data_type=double  read_level=1  write_level=1  ovr_cals=on  view_as=Number  enum_struct={'Disabled', 'Enabled'}  vector_style=Wide Row  use_help_units=on  help='Target fuel pressure delta across injector (rail - manifold)'  units='kPa'  use_header_enum=off  row_header_enum={}  col_header_enum={}  use_min_max=off  min_val=-inf  max_val=inf  use_precision=off  precision=''  gain=1  offset=0  exp=1  use_mototune_group=on  mototune_group=motohawk_vardec_path(gcb)
  motohawk_data_read : MotoHawk_lib/Data Storage Blocks/motohawk_data_read  source=Lookup By Name  structure=Scalar  operation=Read scalar from location by index  sz_vec=4  sz_row=2  sz_col=3  typ=boolean  nam='BankB_Enbl'  checkNull=on  struct_inst_name='MyData'  struct_nam='MyStruct'
  motohawk_data_read1 : MotoHawk_lib/Data Storage Blocks/motohawk_data_read  source=Lookup By Name  structure=Scalar  operation=Read entire data structure at once  sz_vec=4  sz_row=2  sz_col=3  typ=uint8  nam='EngineState'  checkNull=on  struct_inst_name='Struct1'  struct_nam='MyStruct'
  motohawk_fault_def1 : MotoHawk_lib/Fault Management Blocks/motohawk_fault_def  nam='LeanProtect_Fault'  mode=Enabled  id=[]  x=25  y=50  input_suspected=on  indeterminate=off  increment_xy=on  downsample_count=1  ovr_cals=on  ovr_actions=on  show_actions=on  action1_name=''  action1_cond=(None)  action2_name=''  action2_cond=(None)  action3_name=''  action3_cond=(None)  action4_name=''  action4_cond=(None)
  motohawk_fault_status : MotoHawk_lib/Fault Management Blocks/motohawk_fault_status  source=Lookup By Name  nam='Bank1_EquivRatioRangeHigh'  status=Active
  motohawk_fault_status1 : MotoHawk_lib/Fault Management Blocks/motohawk_fault_status  source=Lookup By Name  nam='Bank1_EquivRatioRangeLow'  status=Active
  motohawk_fault_status2 : MotoHawk_lib/Fault Management Blocks/motohawk_fault_status  source=Lookup By Name  nam='Bank2_EquivRatioRangeHigh'  status=Active
  motohawk_fault_status3 : MotoHawk_lib/Fault Management Blocks/motohawk_fault_status  source=Lookup By Name  nam='Bank2_EquivRatioRangeLow'  status=Active
  wires:
  Logical Operator4/1 -> motohawk_fault_def1/1
  Sensors/1 -> Bus Selector4/1, Bus Selector1/1
  Logical Operator3/1 -> Logical Operator4/1
  Logical Operator1/1 -> Logical Operator3/1
  Relational Operator1/1 -> Logical Operator4/2
  Bus Selector4/1 -> Relational Operator1/1  "<O2_BankA>"
  motohawk_fault_status2/1 -> Product/2
  motohawk_fault_status3/1 -> Product1/2
  motohawk_data_read/1 -> Product/1, Product1/1
  Bus Selector1/1 -> Logical Operator1/5  "<ESTOP>"
  motohawk_fault_status1/1 -> Logical Operator1/4
  motohawk_fault_status/1 -> Logical Operator1/3
  Product1/1 -> Logical Operator1/2
  Product/1 -> Logical Operator1/1
  motohawk_calibration3/1 -> Relational Operator1/2
  motohawk_data_read1/1 -> Run State/1
  Run State/1 -> Logical Operator4/3

== system BaseEngineController_LS_112/Foreground/Control/Diagnostics/Low Oil Pressure Fault Logic ==
  Sensors : Inport
  Bus Selector : BusSelector  OutputSignals=RawProcessed.EngineState
  Bus Selector1 : BusSelector  OutputSignals=RawIndexes.RPM09Idx
  Bus Selector4 : BusSelector  OutputSignals=Raw.LinearSensors.OilPres
  Logical Operator1 : Logic  Operator=OR  AllPortsSameDT=off  OutDataTypeStr=boolean
  Logical Operator3 : Logic  Operator=NOT  Inputs=3  AllPortsSameDT=off  OutDataTypeStr=boolean
  Logical Operator4 : Logic  Inputs=3  AllPortsSameDT=off  OutDataTypeStr=boolean
  Relational Operator1 : RelationalOperator  Operator=<  OutDataTypeStr=boolean
  Relational Operator2 : RelationalOperator  Operator=<  OutDataTypeStr=boolean
  Run State : motohawk_control_primitives_lib/CompareTo  SystemSampleTime=-1  op===  val=3
  motohawk_fault_def1 : MotoHawk_lib/Fault Management Blocks/motohawk_fault_def  nam='NoOil_Fault'  mode=Sticky  id=[]  x=1  y=2  input_suspected=on  indeterminate=off  increment_xy=on  downsample_count=1  ovr_cals=on  ovr_actions=on  show_actions=on  action1_name='EngineShutdown'  action1_cond=Active  action2_name=''  action2_cond=(None)  action3_name=''  action3_cond=(None)  action4_name=''  action4_cond=(None)
  motohawk_fault_status : MotoHawk_lib/Fault Management Blocks/motohawk_fault_status  source=Lookup By Name  nam='OilPresRangeHigh'  status=Active
  motohawk_fault_status1 : MotoHawk_lib/Fault Management Blocks/motohawk_fault_status  source=Lookup By Name  nam='OilPresRangeLow'  status=Active
  motohawk_interpolation_1d : MotoHawk_lib/Lookup Tables/motohawk_interpolation_1d  nam='MinOilPressure_Fault'  table_data=[0 10 20 20 30 40 40 50 50]  show_more=on  data_type=Inherit from 'Table Data'  storage=NonAdaptive  read_level=1  write_level=1  ovr_cals=on  use_help=on  help='Minimum oil pressure based on RPM - engine faults and shuts down below this'  units='psi'  use_min_max=off  min_val=-inf  max_val=inf  use_precision=off  precision=''  gain=1  offset=0  exp=1  use_links=off  prelookup_block=''  output_name=''  use_mototune_group=on  mototune_group=motohawk_vardec_path(gcb)
  motohawk_interpolation_1d3 : MotoHawk_lib/Lookup Tables/motohawk_interpolation_1d  nam='MinOilPressure_Warn'  table_data=[20 20 20 20 30 30 40 40 50]  show_more=on  data_type=Inherit from 'Table Data'  storage=NonAdaptive  read_level=1  write_level=1  ovr_cals=on  use_help=on  help='Minimum oil pressure based on RPM - indicator light comes on below this'  units='psi'  use_min_max=off  min_val=-inf  max_val=inf  use_precision=off  precision=''  gain=1  offset=0  exp=1  use_links=off  prelookup_block=''  output_name=''  use_mototune_group=on  mototune_group=motohawk_vardec_path(gcb)
  LowOilPres : Outport
  wires:
  Logical Operator4/1 -> motohawk_fault_def1/1
  Sensors/1 -> Bus Selector/1, Bus Selector4/1, Bus Selector1/1
  Logical Operator3/1 -> Logical Operator4/1
  Logical Operator1/1 -> Logical Operator3/1
  motohawk_fault_status1/1 -> Logical Operator1/2
  motohawk_fault_status/1 -> Logical Operator1/1
  Bus Selector/1 -> Run State/1  "<EngineState>"
  Relational Operator1/1 -> LowOilPres/1
  motohawk_interpolation_1d3/1 -> Relational Operator1/2
  Bus Selector1/1 -> motohawk_interpolation_1d/1, motohawk_interpolation_1d3/1  "<RPM09Idx>"
  motohawk_interpolation_1d/1 -> Relational Operator2/2
  Bus Selector4/1 -> Relational Operator2/1, Relational Operator1/1  "<OilPres>"
  Run State/1 -> Logical Operator4/2
  Relational Operator2/1 -> Logical Operator4/3

== system BaseEngineController_LS_112/Foreground/Control/Diagnostics/Low Voltage ==
  Sensors : Inport
  Bus Selector4 : BusSelector  OutputSignals=Raw.LinearSensors.SysVolt
  Logical Operator : Logic  Operator=OR  AllPortsSameDT=off  OutDataTypeStr=boolean
  Logical Operator1 : Logic  Operator=NOT  Inputs=3  AllPortsSameDT=off  OutDataTypeStr=boolean
  Logical Operator2 : Logic  Inputs=3  AllPortsSameDT=off  OutDataTypeStr=boolean
  Logical Operator3 : Logic  Operator=OR  AllPortsSameDT=off  OutDataTypeStr=boolean
  Logical Operator4 : Logic  Inputs=3  AllPortsSameDT=off  OutDataTypeStr=boolean
  Logical Operator5 : Logic  Inputs=3  AllPortsSameDT=off  OutDataTypeStr=boolean
  Relational Operator : RelationalOperator  Operator=<=  OutDataTypeStr=boolean
  Relational Operator1 : RelationalOperator  OutDataTypeStr=boolean
  Relational Operator2 : RelationalOperator  Operator=<=  OutDataTypeStr=boolean
  Run State : motohawk_control_primitives_lib/CompareTo  SystemSampleTime=-1  op===  val=3
  Run State1 : motohawk_control_primitives_lib/CompareTo  SystemSampleTime=-1  op===  val=3
  Run State2 : motohawk_control_primitives_lib/CompareTo  SystemSampleTime=-1  op===  val=3
  Run State3 : motohawk_control_primitives_lib/CompareTo  SystemSampleTime=-1  op===  val=2
  motohawk_calibration : MotoHawk_lib/Calibration & Probing Blocks/motohawk_calibration  nam='LVDiag_AltInop'  val=12  storage=Calibration  show_more=off  name_source=Use Parameter  data_type=Inherit from 'Default Value'  read_level=1  write_level=1  ovr_cals=on  view_as=Number  enum_struct={'Disabled', 'Enabled'}  vector_style=Wide Row  use_help_units=off  help=''  units=''  use_header_enum=off  row_header_enum={}  col_header_enum={}  use_min_max=off  min_val=-inf  max_val=inf  use_precision=off  precision=''  gain=1  offset=0  exp=1  use_mototune_group=off  mototune_group=motohawk_vardec_path(gcb)
  motohawk_calibration1 : MotoHawk_lib/Calibration & Probing Blocks/motohawk_calibration  nam='LVDiag_VoltTooHigh'  val=15  storage=Calibration  show_more=off  name_source=Use Parameter  data_type=Inherit from 'Default Value'  read_level=1  write_level=1  ovr_cals=on  view_as=Number  enum_struct={'Disabled', 'Enabled'}  vector_style=Wide Row  use_help_units=off  help=''  units=''  use_header_enum=off  row_header_enum={}  col_header_enum={}  use_min_max=off  min_val=-inf  max_val=inf  use_precision=off  precision=''  gain=1  offset=0  exp=1  use_mototune_group=off  mototune_group=motohawk_vardec_path(gcb)
  motohawk_calibration2 : MotoHawk_lib/Calibration & Probing Blocks/motohawk_calibration  nam='LVDiag_VoltLow'  val=11  storage=Calibration  show_more=off  name_source=Use Parameter  data_type=Inherit from 'Default Value'  read_level=1  write_level=1  ovr_cals=on  view_as=Number  enum_struct={'Disabled', 'Enabled'}  vector_style=Wide Row  use_help_units=off  help=''  units=''  use_header_enum=off  row_header_enum={}  col_header_enum={}  use_min_max=off  min_val=-inf  max_val=inf  use_precision=off  precision=''  gain=1  offset=0  exp=1  use_mototune_group=off  mototune_group=motohawk_vardec_path(gcb)
  motohawk_data_read1 : MotoHawk_lib/Data Storage Blocks/motohawk_data_read  source=Lookup By Name  structure=Scalar  operation=Read entire data structure at once  sz_vec=4  sz_row=2  sz_col=3  typ=uint8  nam='EngineState'  checkNull=on  struct_inst_name='Struct1'  struct_nam='MyStruct'
  motohawk_data_read2 : MotoHawk_lib/Data Storage Blocks/motohawk_data_read  source=Lookup By Name  structure=Scalar  operation=Read entire data structure at once  sz_vec=4  sz_row=2  sz_col=3  typ=uint8  nam='EngineState'  checkNull=on  struct_inst_name='Struct1'  struct_nam='MyStruct'
  motohawk_data_read3 : MotoHawk_lib/Data Storage Blocks/motohawk_data_read  source=Lookup By Name  structure=Scalar  operation=Read entire data structure at once  sz_vec=4  sz_row=2  sz_col=3  typ=uint8  nam='EngineState'  checkNull=on  struct_inst_name='Struct1'  struct_nam='MyStruct'
  motohawk_fault_def1 : MotoHawk_lib/Fault Management Blocks/motohawk_fault_def  nam='AltInop_Fault'  mode=Enabled  id=[]  x=25  y=50  input_suspected=on  indeterminate=off  increment_xy=on  downsample_count=1  ovr_cals=on  ovr_actions=on  show_actions=on  action1_name=''  action1_cond=(None)  action2_name=''  action2_cond=(None)  action3_name=''  action3_cond=(None)  action4_name=''  action4_cond=(None)
  motohawk_fault_def2 : MotoHawk_lib/Fault Management Blocks/motohawk_fault_def  nam='VoltTooHigh_Fault'  mode=Enabled  id=[]  x=25  y=50  input_suspected=on  indeterminate=off  increment_xy=on  downsample_count=1  ovr_cals=on  ovr_actions=on  show_actions=on  action1_name=''  action1_cond=(None)  action2_name=''  action2_cond=(None)  action3_name=''  action3_cond=(None)  action4_name=''  action4_cond=(None)
  motohawk_fault_def3 : MotoHawk_lib/Fault Management Blocks/motohawk_fault_def  nam='VoltLow_Fault'  mode=Enabled  id=[]  x=25  y=50  input_suspected=on  indeterminate=off  increment_xy=on  downsample_count=1  ovr_cals=on  ovr_actions=on  show_actions=on  action1_name=''  action1_cond=(None)  action2_name=''  action2_cond=(None)  action3_name=''  action3_cond=(None)  action4_name=''  action4_cond=(None)
  motohawk_fault_status1 : MotoHawk_lib/Fault Management Blocks/motohawk_fault_status  source=Lookup By Name  nam='SysVoltRangeHigh'  status=Active
  motohawk_fault_status4 : MotoHawk_lib/Fault Management Blocks/motohawk_fault_status  source=Lookup By Name  nam='SysVoltRangeLow'  status=Active
  wires:
  Sensors/1 -> Bus Selector4/1
  motohawk_data_read1/1 -> Run State/1
  Run State/1 -> Logical Operator4/3
  motohawk_fault_status1/1 -> Logical Operator3/1
  Logical Operator3/1 -> Logical Operator1/1
  motohawk_fault_status4/1 -> Logical Operator3/2
  Bus Selector4/1 -> Relational Operator/1, Relational Operator1/1, Relational Operator2/1  "<SysVolt>"
  Relational Operator/1 -> Logical Operator4/2
  motohawk_calibration/1 -> Relational Operator/2
  Logical Operator1/1 -> Logical Operator4/1, Logical Operator2/1, Logical Operator5/1
  motohawk_data_read2/1 -> Run State1/1
  Run State1/1 -> Logical Operator2/3
  Relational Operator1/1 -> Logical Operator2/2
  motohawk_calibration1/1 -> Relational Operator1/2
  Logical Operator4/1 -> motohawk_fault_def1/1
  Logical Operator2/1 -> motohawk_fault_def2/1
  motohawk_data_read3/1 -> Run State2/1, Run State3/1
  Relational Operator2/1 -> Logical Operator5/2
  motohawk_calibration2/1 -> Relational Operator2/2
  Logical Operator5/1 -> motohawk_fault_def3/1
  Run State2/1 -> Logical Operator/1
  Run State3/1 -> Logical Operator/2
  Logical Operator/1 -> Logical Operator5/3
